simulink library "INT_TClntDspl_DD"  (R2016b)
settings: Solver=VariableStepAuto  StartTime=0.0  StopTime=10.0  RelTol=1e-3
settings Model: Creator=Wei Liang  LastModifiedBy=Wei Liang

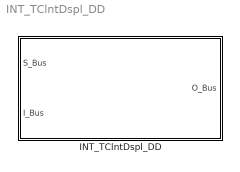
== system INT_TClntDspl_DD ==
  INT_TClntDspl_DD : Subsystem

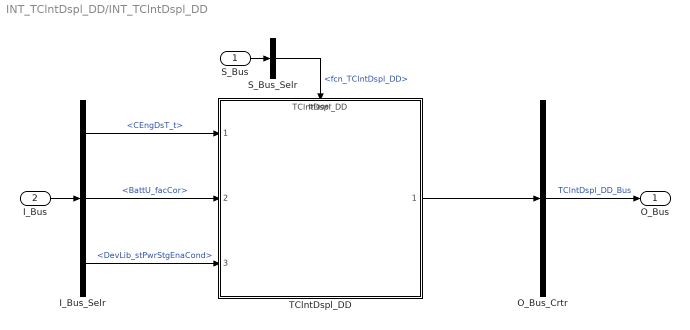
== system INT_TClntDspl_DD/INT_TClntDspl_DD ==
  S_Bus : Inport
  I_Bus : Inport  Port=2
  I_Bus_Selr : BusSelector  OutputSignals=CEngDsT_t,BattU_facCor,DevLib_stPwrStgEnaCond
  O_Bus_Crtr : BusCreator  Inputs=1
  S_Bus_Selr : BusSelector  OutputSignals=fcn_TClntDspl_DD
  TClntDspl_DD : ModelReference  ModelNameDialog=TClntDspl_DD  SimulationMode=Normal  ModelReferenceVersion=1.17  TriggerPortName=function  TriggerPortTriggerType=function-call  TriggerPortStatesWhenEnabling=held
  O_Bus : Outport
  wires:
  S_Bus_Selr/1 -> TClntDspl_DD/Trigger  "<fcn_TClntDspl_DD>"
  S_Bus/1 -> S_Bus_Selr/1
  I_Bus/1 -> I_Bus_Selr/1
  I_Bus_Selr/1 -> TClntDspl_DD/1  "<CEngDsT_t>"
  I_Bus_Selr/2 -> TClntDspl_DD/2  "<BattU_facCor>"
  I_Bus_Selr/3 -> TClntDspl_DD/3  "<DevLib_stPwrStgEnaCond>"
  O_Bus_Crtr/1 -> O_Bus/1  "TClntDspl_DD_Bus"
  TClntDspl_DD/1 -> O_Bus_Crtr/1
